simulink model "Appl_DrComfort_CtrlModel"  (R2018b)
settings: configuration reference "CodeConfig_10_ms" (kept outside this file)
undefined symbols (not defined in the file): D_Active, D_CLOSE, D_Inactive, D_InitDelayTime, D_OPEN, D_SoftDistanceDrLegnth, D_WelcomeDistance, FALSE, TRUE
libraries: DareLib x50, simulink x1
(part 2 of 2)

== stateflow chart Appl_DrComfort_CtrlModel/UpDataInputInfo/InputSignalProcess/WelcomePrecondition_Trigger/Precondition_Trigger ==
  state CommonCondition [parallel]
    settings: executionOrder=1
    state CommonInit
      en:
      CommonFlag = FALSE;
      WelcomeStopReason = ...
      enWelStopCause.EN_WelStop_VoltageError;
    state CommonActive
      en:
      CommonFlag = TRUE;
    state CommonInactive
      en:
      CommonFlag = FALSE;
    (default) -> CommonInit
    CommonInit -> CommonActive [order 1] : /*迎宾使能 && 无纵向堵转故障 && 无纵向继电器粘连故障
        | && 无靠背堵转故障 && 无靠背继电器粘连故障&& 无busoff故障
        | && PN档 && 座椅纵向已学习 &&无高优先级运动 && 电压正常 && 不处于小憩模式开启状态*/
        | [TRUE == ComfortOpenFlag ...
        | && FALSE == MtrWel_LengthLockSts ...
        | && FALSE == MtrWel_LengthRelayFaultSts ...
        | && FALSE == MtrWel_BackLockSts ...
        | && FALSE == MtrWel_BackRelayFaultSts ...
        | && FALSE == MtrWel_BusoffFlag ...
        | && TRUE == Gear_PN_Flag ...
        | && TRUE == SeatLearnResult ...
        | && enSeatMotorRunType.EN_ComfortEnable >= MtrWel_CurrentMoveType ...
        | && FALSE == MtrWel_0x28E_BDCLostFlag ...
        | && enFinalPowerMode.EN_NORMAL_VOLT == MtrWel_VoltMode ...
        | && TRUE == MtrWel_VoltSatisfy ...
        | && enNapMode.EN_NapMode_Open != MtrWel_NapMode]
        | /WelcomeStopReason = enWelStopCause.EN_WelStop_NULL;
    CommonInactive -> CommonActive : /*迎宾使能 && 无纵向堵转故障 && 无纵向继电器粘连故障
        | && 无靠背堵转故障 && 无靠背继电器粘连故障&& 无busoff故障
        | && PN档 && 座椅纵向已学习 &&无高优先级运动 && 电压正常 && 不处于小憩模式开启状态*/
        | [TRUE == ComfortOpenFlag ...
        | && FALSE == MtrWel_LengthLockSts ...
        | && FALSE == MtrWel_LengthRelayFaultSts ...
        | && FALSE == MtrWel_BackLockSts ...
        | && FALSE == MtrWel_BackRelayFaultSts ...
        | && FALSE == MtrWel_BusoffFlag ...
        | && TRUE == Gear_PN_Flag ...
        | && TRUE == SeatLearnResult ...
        | && enSeatMotorRunType.EN_ComfortEnable >= MtrWel_CurrentMoveType ...
        | && FALSE == MtrWel_0x28E_BDCLostFlag ...
        | && enFinalPowerMode.EN_NORMAL_VOLT == MtrWel_VoltMode ...
        | && TRUE == MtrWel_VoltSatisfy ...
        | && enNapMode.EN_NapMode_Open != MtrWel_NapMode]
        | /WelcomeStopReason = enWelStopCause.EN_WelStop_NULL;
    CommonInit -> CommonInactive [order 2] : /*迎宾禁能*/
        | [TRUE != ComfortOpenFlag]
        | /WelcomeStopReason = enWelStopCause.EN_WelStop_PRM;
        | //Set_WelcomeUpdatePosiFlag(TRUE);
    CommonActive -> CommonInactive [order 1] : /*迎宾禁能*/
        | [TRUE != ComfortOpenFlag]
        | /WelcomeStopReason = enWelStopCause.EN_WelStop_PRM;
        | Set_WelcomeUpdatePosiFlag(TRUE);
    CommonInit -> CommonInactive [commented out] : /*有纵向霍尔故障*/
        | [FALSE != MtrWel_LengthHallFaultSts]
        | /WelcomeStopReason = enWelStopCause.EN_WelStop_HallFault
    CommonActive -> CommonInactive [commented out] : /*有纵向霍尔故障*/
        | [FALSE != MtrWel_LengthHallFaultSts]
        | /WelcomeStopReason = enWelStopCause.EN_WelStop_HallFault
    CommonInit -> CommonInactive [order 3] : /*有纵向或靠背堵转故障*/
        | [FALSE != MtrWel_LengthLockSts || FALSE != MtrWel_BackLockSts]
        | /WelcomeStopReason = enWelStopCause.EN_WelStop_LockFault;
        | //Set_WelcomeUpdatePosiFlag(TRUE);
    CommonActive -> CommonInactive [order 2] : /*有纵向或靠背堵转故障*/
        | [FALSE != MtrWel_LengthLockSts || FALSE != MtrWel_BackLockSts]
        | /WelcomeStopReason = enWelStopCause.EN_WelStop_LockFault;
        | Set_WelcomeUpdatePosiFlag(TRUE);
    CommonInit -> CommonInactive [order 4] : /*存在纵向或靠背继电器故障*/
        | [FALSE != MtrWel_LengthRelayFaultSts ...
        | || FALSE != MtrWel_BackRelayFaultSts]
        | /WelcomeStopReason = enWelStopCause.EN_WelStop_RelayFault
    CommonActive -> CommonInactive [order 3] : /*存在纵向或靠背继电器故障*/
        | [FALSE != MtrWel_LengthRelayFaultSts...
        | || FALSE != MtrWel_BackRelayFaultSts]
        | /WelcomeStopReason = enWelStopCause.EN_WelStop_RelayFault
    CommonInit -> CommonInactive [order 5] : /*有busoff故障*/
        | [FALSE != MtrWel_BusoffFlag]
        | /WelcomeStopReason = enWelStopCause.EN_WelStop_Busoff
    CommonActive -> CommonInactive [order 4] : /*有busoff故障*/
        | [FALSE != MtrWel_BusoffFlag]
        | /WelcomeStopReason = enWelStopCause.EN_WelStop_Busoff
    CommonInit -> CommonInactive [order 6] : /*非PN档*/
        | [TRUE != Gear_PN_Flag]
        | /WelcomeStopReason = enWelStopCause.EN_WelStop_enNotGearPN
    CommonActive -> CommonInactive [order 5] : /*非PN档*/
        | [TRUE != Gear_PN_Flag]
        | /WelcomeStopReason = enWelStopCause.EN_WelStop_enNotGearPN
    CommonInit -> CommonInactive [order 7] : /*纵向或靠背未学习*/
        | [TRUE != SeatLearnResult]
        | /WelcomeStopReason = enWelStopCause.EN_WelStop_enNotLearn;
        | //Set_WelcomeUpdatePosiFlag(TRUE);
    CommonActive -> CommonInactive [order 6] : /*纵向或靠背未学习*/
        | [TRUE != SeatLearnResult]
        | /WelcomeStopReason = enWelStopCause.EN_WelStop_enNotLearn;
        | Set_WelcomeUpdatePosiFlag(TRUE);
    CommonInit -> CommonInactive [order 8] : /*有高由于迎宾运动的请求*/
        | [enSeatMotorRunType.EN_ComfortEnable < MtrWel_CurrentMoveType]
        | /WelcomeStopReason = enWelStopCause.EN_WelStop_OtherMove;
        | //Set_WelcomeUpdatePosiFlag(TRUE);
    CommonActive -> CommonInactive [order 7] : /*有高由于迎宾运动的请求*/
        | [enSeatMotorRunType.EN_ComfortEnable < MtrWel_CurrentMoveType]
        | /WelcomeStopReason = enWelStopCause.EN_WelStop_OtherMove;
        | Set_WelcomeUpdatePosiFlag(TRUE);
    CommonInit -> CommonInactive [order 9] : /*门信号丢失*/
        | [TRUE == MtrWel_0x28E_BDCLostFlag]
        | /WelcomeStopReason = enWelStopCause.EN_WelStop_enBDCDoorLost
    CommonActive -> CommonInactive [order 8] : /*门信号丢失*/
        | [TRUE == MtrWel_0x28E_BDCLostFlag]
        | /WelcomeStopReason = enWelStopCause.EN_WelStop_enBDCDoorLost
    CommonInit -> CommonInactive [order 10] : /*电压非正常模式*/
        | [enFinalPowerMode.EN_NORMAL_VOLT != MtrWel_VoltMode ...
        | || TRUE != MtrWel_VoltSatisfy]
        | /WelcomeStopReason = enWelStopCause.EN_WelStop_VoltageError
    CommonActive -> CommonInactive [order 9] : /*电压非正常模式*/
        | [enFinalPowerMode.EN_NORMAL_VOLT != MtrWel_VoltMode ...
        | || TRUE != MtrWel_VoltSatisfy]
        | /WelcomeStopReason = enWelStopCause.EN_WelStop_VoltageError
    CommonInit -> CommonInactive [order 11] : /*处于小憩模式开启状态*/
        | [enNapMode.EN_NapMode_Open == MtrWel_NapMode]
        | /WelcomeStopReason = enWelStopCause.EN_WelStop_NapMode
    CommonActive -> CommonInactive [order 10] : /*处于小憩模式开启状态*/
        | [enNapMode.EN_NapMode_Open == MtrWel_NapMode]
        | /WelcomeStopReason = enWelStopCause.EN_WelStop_NapMode
  state UpdatePosi [parallel]
    settings: executionOrder=3
    (default) -> (junction 167)
    UpdatePosi -> (junction 167)
    (junction 167) -> (junction 170)
    (junction 170) -> (junction 172) [order 1] : /* 纵向坐标变化 且非舒适功能调节 需要更新纵向位置 */
        | [enSeatMotorRunType.EN_ComfortEnable != MtrWel_CurrentMoveType ...
        | && enSeatMotorRunType.EN_NULL != MtrWel_CurrentMoveType ...
        | && (hasChangedTo(MtrWel_LengthCmd,1) || hasChangedTo(MtrWel_LengthCmd,2))]
    (junction 170) -> (junction 176) [order 2]
    (junction 172) -> (junction 174) : {Set_WelcomeUpdatePosiFlag(TRUE);}
    (junction 174) -> (junction 176)
    (junction 176) -> (junction 179)
  state Set_WelcomeUpdatePosiFlag(In1) [function]
  state DoorSts [parallel]
    settings: executionOrder=2
    state DoorInit
      en:
      WaitTimeCnt = 0;
      LocalDoorSts = 0xFF;
      du:
      WaitTimeCnt += 1;
      LocalDoorSts = Get_DoorSts();
      ex:
      WaitTimeCnt = 0;
      LocalDoorSts = Get_DoorSts();
    state DoorSts
      du:
      LocalDoorSts = MtrWel_BDC_FLDoorSts;
      E2pDoorSts = Get_DoorSts();
      state BackwardTriggerCondition [parallel]
        settings: executionOrder=1
        state BWActive
          en:
          BackwardTriggerCondition = TRUE;
        state BWInactive
          en:
          BackwardTriggerCondition = FALSE;
        (default) -> BWInactive
        BWInactive -> BWActive : /* 迎宾后移条件
            | C5、左前车门状态由关闭→打开（BDC_FLDoorSts=0x0:Close→0x1:Open）且前数据正常*/
            | [hasChangedTo(LocalDoorSts,D_OPEN) ...
            | && E2pDoorSts <= D_OPEN]
        BWActive -> BWInactive : /*2个运行周期*/
            | after(2,tick)
      state Change [parallel]
        settings: executionOrder=3
        Change -> (junction 149)
        (junction 149) -> (junction 154)
        (junction 154) -> (junction 156) [order 1] : /* 门状态变化 存数据 */
            | [hasChanged(LocalDoorSts) && LocalDoorSts <= D_OPEN]
        (junction 154) -> (junction 160) [order 2]
        (junction 156) -> (junction 158) : {Set_DoorSts(LocalDoorSts);}
        (junction 158) -> (junction 160)
        (junction 160) -> (junction 163)
      state ForwardTriggercondition [parallel]
        settings: executionOrder=2
        state FWInactive
          en:
          ForwardTriggerCondition = FALSE;
        state FWActive
          en:
          ForwardTriggerCondition = TRUE;
        (default) -> FWInactive
        FWInactive -> FWActive : /* 迎宾前移条件
            | C6、左前车门状态由打开→关闭（BDC_FLDoorSts=0x1:Open→0x0:Close）且前数据正常*/
            | [hasChangedTo(LocalDoorSts,D_CLOSE)...
            | && E2pDoorSts <= D_OPEN]
        FWActive -> FWInactive : /*2个运行周期*/
            | after(2,tick)
    (default) -> DoorInit
    DoorInit -> DoorSts.DoorSts : /* 等待读取e2p数据 */
        | [WaitTimeCnt > 20]
  state Set_DoorSts(In1) [function]
  state Out1 = Get_DoorSts [function]
  data: In1 function_input; In1 function_input; Out1 function_output; ComfortOpenFlag input; Gear_PN_Flag input; MtrWel_LengthLockSts input; MtrWel_BusoffFlag input; FALSE parameter; TRUE parameter; BackwardTriggerCondition output uint8; ForwardTriggerCondition output uint8; WelcomeStopReason output Enum: enWelStopCause =enWelStopCause.EN_WelStop_VoltageError; MtrWel_CurrentMoveType input; SeatLearnResult input; MtrWel_LengthRelayFaultSts input; MtrWel_0x28E_BDCLostFlag input; MtrWel_VoltMode input; D_CLOSE parameter; D_OPEN parameter; MtrWel_BDC_FLDoorSts input; CommonFlag local uint8; MtrWel_NapMode input; MtrWel_VoltSatisfy input; MtrWel_BackHallFaultSts input; MtrWel_BackRelayFaultSts input; MtrWel_BackLockSts input; WaitTimeCnt local uint8; LocalDoorSts local uint8; MtrWel_LengthCmd input; E2pDoorSts local uint8

== stateflow chart Appl_DrComfort_CtrlModel/UpDataInputInfo/InputSignalProcess/WelcomePRM/ComfortDeal ==
  state SetComfortPrm(in) [function]
  state Init
    en:
    InitTimer = 1;
    ComfortOpenFlag = FALSE;
    ComfortOpenMsg = TRUE;
    du:
    InitTimer ++;
    ex:
    InitTimer = 0;
  state Configurable
    state Enable
      en:
      ComfortOpenFlag = TRUE;
      /**ComfortOpenMsg 报文发送变量****************ComfortOpenFlag迎宾功能是否开启变量即PC1迎宾功能处于开启状态*/
      SetComfortPrm(TRUE);
      ComfortOpenMsg = TRUE;
    state Disable
      en:
      ComfortOpenFlag = FALSE;
      SetComfortPrm(FALSE);
      ComfortOpenMsg = FALSE;
    (junction 38) -> Enable [order 1] : [MtrWel_WelcomeSwitch == 1]
    Enable -> Disable : /*当IVI_St_FLSeatmeet=0x2:Close时，座椅调节舒适进入禁能*/
        | [2 == MtrWel_0x351_IVI_St_FLSeatmeet]
    Disable -> Enable : /*当IVI_St_FLSeatmeet=0x1:Open时，座椅调节舒适进入使能*/
        | [1 == MtrWel_0x351_IVI_St_FLSeatmeet]
    (default) -> (junction 38)
    (junction 38) -> Disable [order 2]
  (default) -> Init
  Init -> Configurable : /*EEPROM迎宾为使能&&座椅电动调节&&P20车型&&初始化完成&&正常电压*/
      | [TRUE == MtrWel_WelcomeEnable ...
      | && (enDrAdjustEnable.EN_DrSixWayMotor == MtrWel_AdjustEnable ...
      | || enDrAdjustEnable.EN_DrTwelveWayMotor == MtrWel_AdjustEnable) ...
      | && enVehTypePrm.enP20 == MtrWel_VehiclePrm ...
      | && InitTimer > D_InitDelayTime ...
      | && enFinalPowerMode.EN_NORMAL_VOLT == MtrWel_VoltMode]
  Configurable -> Init [order 1] : /*恢复出厂设置*/
      | [TRUE == MtrWel_GetRecoverDefaultFlag]
      | /SetComfortPrm(TRUE);
  Configurable -> Init [order 2] : /*((迎宾禁能 || 座椅非6&&12项调节 || 电压非正常模式)&&P20车型)
      | || 非P20车型*/
      | [((TRUE != MtrWel_WelcomeEnable ...
      | || (enDrAdjustEnable.EN_DrSixWayMotor != MtrWel_AdjustEnable ...
      | && enDrAdjustEnable.EN_DrTwelveWayMotor != MtrWel_AdjustEnable) ...
      | || enFinalPowerMode.EN_NORMAL_VOLT != MtrWel_VoltMode) ...
      | && enVehTypePrm.enP20 == MtrWel_VehiclePrm) ...
      | || enVehTypePrm.enP20 != MtrWel_VehiclePrm]
  data: in function_input; MtrWel_0x351_IVI_St_FLSeatmeet input; MtrWel_WelcomeEnable input; ComfortOpenFlag output uint8; TRUE parameter; FALSE parameter; InitTimer local uint8; MtrWel_VoltMode input; MtrWel_AdjustEnable input; MtrWel_VehiclePrm input; MtrWel_WelcomeSwitch input; D_InitDelayTime parameter; MtrWel_GetRecoverDefaultFlag input; ComfortOpenMsg output uint8
